simulink model "test_diff"  (R2020b)
settings: Solver=FixedStepAuto  StartTime=0.0  StopTime=20  FixedStep=0.1  RelTol=1e-3
model workspace (MATLAB code in the model file):
  | R = 0.266;
  | r = 0.04;
  | a = 0.3;
  | b = 0.8;
  | anpha1 = -pi/2;
  | anpha2 = pi/6;
  | anpha3 = 5*pi/6;
  | m1 = 0.42;
  | m2 = 0.2;
  | m3 = 0.75;
  | IAy = m1*a*a/3;
  | g = 9.81;
settings Model: OrderedModelArguments=off  Creator=ShiningDanyang  LastModifiedBy=ShiningDanyang

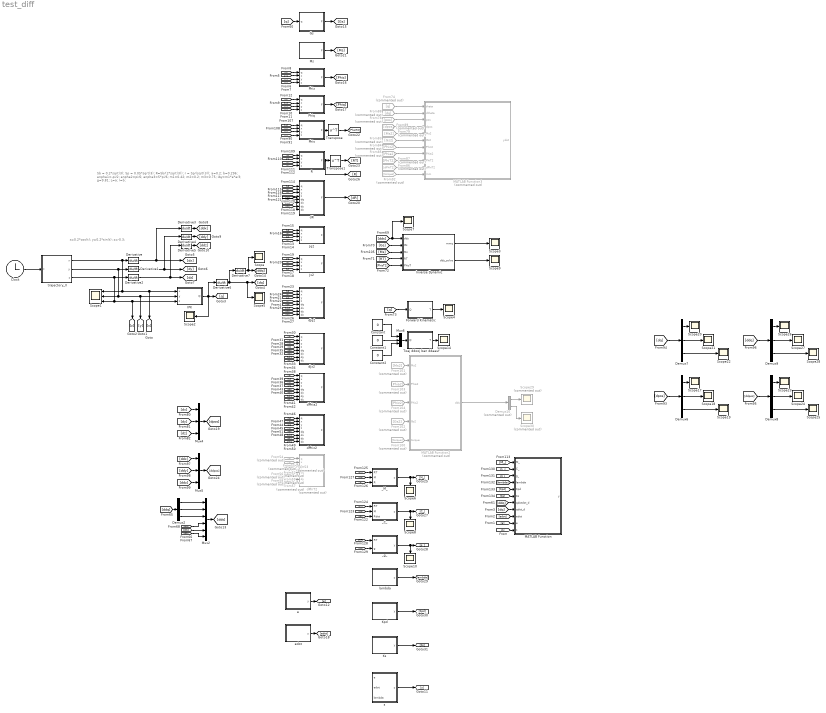
== system test_diff ==
  note: x=0.2*cos(t); y=0.2*sin(t); z=-0.3;
  note: Sb = 0.2*sqrt(3); Sp = 0.05*sqrt(3);
      | R=Sb/(2*sqrt(3)); r = Sp/(sqrt(3));
      | a=0.2; b=0.296;
      | anpha1=-pi/2; anpha2=pi/6; anpha3=5*pi/6;
      | m1=0.42; m2=0.2; m3=0.75;
      | IAy=m1*a*a/3; g=9.81;
      | L=a; l=b;
  Clock : Clock
  Constant : Constant  Value=0
  Constant1 : Constant  Value=0
  Constant2 : Constant  Value=0
  Demux10 : Demux  Commented=on  Outputs=2
  Demux{2,6..9} (5 alike) : Demux  Outputs=3
  Derivative{,1..7} (8 alike) : Derivative
  Forward Kinematic : MATLAB Function  TreatAsAtomicUnit=on
  From100 : From  Commented=on  GotoTag=torque
  From101 : From  Commented=on  GotoTag=Ms2
  From102 : From  Commented=on  GotoTag=Gs2
  From103 : From  Commented=on  GotoTag=Phia2
  From104 : From  Commented=on  GotoTag=Phiz2
  From52 : From  Commented=on  GotoTag=y
  From53 : From  Commented=on  GotoTag=z
  From54 : From  Commented=on  GotoTag=q
  From55 : From  Commented=on  GotoTag=x
  From56 : From  Commented=on  GotoTag=dx
  From57 : From  Commented=on  GotoTag=dy
  From58 : From  Commented=on  GotoTag=dz
  From59 : From  Commented=on  GotoTag=dq
  From74 : From  Commented=on  GotoTag=q
  From78 : From  Commented=on  GotoTag=pos
  From79 : From  Commented=on  GotoTag=Ms2
  From83 : From  Commented=on  GotoTag=Gs2
  From84 : From  Commented=on  GotoTag=Phiz2
  From85 : From  Commented=on  GotoTag=Phia2
  From86 : From  Commented=on  GotoTag=dPhiT2
  From87 : From  Commented=on  GotoTag=PhiT2
  From88 : From  Commented=on  GotoTag=dq
  From89 : From  Commented=on  GotoTag=dpos
  From92 : From  Commented=on  GotoTag=torque
  Gs : MATLAB Function  TreatAsAtomicUnit=on
  IPK : MATLAB Function  TreatAsAtomicUnit=on
  "Inverse Dynamic " : MATLAB Function  TreatAsAtomicUnit=on
  Jq2 : MATLAB Function  TreatAsAtomicUnit=on
  Jx2 : MATLAB Function  TreatAsAtomicUnit=on
  Kpd : MATLAB Function  TreatAsAtomicUnit=on
  Ks : MATLAB Function  TreatAsAtomicUnit=on
  MATLAB Function : MATLAB Function  TreatAsAtomicUnit=on
  MATLAB Function2 : MATLAB Function  Commented=on  TreatAsAtomicUnit=on
  MATLAB Function3 : MATLAB Function  Commented=on  TreatAsAtomicUnit=on
  Ms : MATLAB Function  TreatAsAtomicUnit=on
  Mux2 : Mux  Inputs=6
  Mux4 : Mux  Inputs=3
  Mux5 : Mux  Inputs=3
  Mux6 : Mux  Inputs=3
  Phiq : MATLAB Function  TreatAsAtomicUnit=on
  Phis : MATLAB Function  TreatAsAtomicUnit=on
  Phiz : MATLAB Function  TreatAsAtomicUnit=on
  R : MATLAB Function  TreatAsAtomicUnit=on
  Scope{,2..10,14,17..28} (23 alike) : Scope
  Scope1 : Scope  NumInputPorts=3
  Scope29 : Scope  Commented=on
  Scope30 : Scope  Commented=on
  Toaj ddooj ban ddaauf : MATLAB Function  TreatAsAtomicUnit=on
  Transpose : Math  Operator=transpose  SaturateOnIntegerOverflow=on
  Transpose1 : Math  Operator=transpose  SaturateOnIntegerOverflow=on
  _C_ : MATLAB Function  TreatAsAtomicUnit=on
  _M_ : MATLAB Function  TreatAsAtomicUnit=on
  _g_ : MATLAB Function  TreatAsAtomicUnit=on
  dJq2 : MATLAB Function  TreatAsAtomicUnit=on
  dJx2 : MATLAB Function  TreatAsAtomicUnit=on
  dPhiT2 : MATLAB Function  Commented=on  TreatAsAtomicUnit=on
  dPhia2 : MATLAB Function  TreatAsAtomicUnit=on
  dPhiz2 : MATLAB Function  TreatAsAtomicUnit=on
  dR : MATLAB Function  TreatAsAtomicUnit=on
  e : MATLAB Function  TreatAsAtomicUnit=on
  edot : MATLAB Function  TreatAsAtomicUnit=on
  lambda : MATLAB Function  TreatAsAtomicUnit=on
  s : MATLAB Function  TreatAsAtomicUnit=on
  trajectory_X : MATLAB Function  TreatAsAtomicUnit=on
  wires:
  Clock/1 -> trajectory_X/1(t)
  trajectory_X/1(x) -> IPK/1(x), [x], Scope1/1, Derivative/1
  trajectory_X/2(y) -> IPK/2(y), [y], Scope1/2, Derivative1/1
  trajectory_X/3(z) -> IPK/3(z), [z], Scope1/3, Derivative2/1
  Derivative2/1 -> [dz], Derivative5/1
  Derivative1/1 -> [dy], Derivative4/1
  Derivative/1 -> [dx], Derivative3/1
  IPK/1(Q) -> Scope2/1, [q], Derivative6/1
  Derivative6/1 -> Derivative7/1, Scope5/1, [dq]
  [q] -> Phiz/1(q)
  [x] -> Phiz/2(x)
  [y] -> Phiz/3(y)
  [z] -> Phiz/4(z)
  [z] -> Phiq/4(z)
  [y] -> Phiq/3(y)
  [x] -> Phiq/2(x)
  [q] -> Phiq/1(q)
  [y] -> Jx2/3(y)
  [q] -> Jx2/1(q)
  [x] -> Jx2/2(x)
  [z] -> Jx2/4(z)
  [q] -> dJq2/1(q)
  [x] -> dJq2/2(x)
  [y] -> dJq2/3(y)
  [z] -> dJq2/4(z)
  [dx] -> dJq2/6(dx)
  [dy] -> dJq2/7(dy)
  [dz] -> dJq2/8(dz)
  [dq] -> dJq2/5(dq)
  [z] -> dJx2/4(z)
  [dx] -> dJx2/6(dx)
  [x] -> dJx2/2(x)
  [dq] -> dJx2/5(dq)
  [y] -> dJx2/3(y)
  [dy] -> dJx2/7(dy)
  [dz] -> dJx2/8(dz)
  [q] -> dJx2/1(q)
  [z] -> dPhia2/4(z)
  [dx] -> dPhia2/6(dx)
  [x] -> dPhia2/2(x)
  [dq] -> dPhia2/5(dq)
  [y] -> dPhia2/3(y)
  [dy] -> dPhia2/7(dy)
  [dz] -> dPhia2/8(dz)
  [q] -> dPhia2/1(q)
  [z] -> dPhiz2/4(z)
  [dx] -> dPhiz2/6(dx)
  [x] -> dPhiz2/2(x)
  [dq] -> dPhiz2/5(dq)
  [y] -> dPhiz2/3(y)
  [dy] -> dPhiz2/7(dy)
  [dz] -> dPhiz2/8(dz)
  [q] -> dPhiz2/1(q)
  From53/1 -> dPhiT2/4(z)
  From56/1 -> dPhiT2/6(dx)
  From55/1 -> dPhiT2/2(x)
  From59/1 -> dPhiT2/5(dq)
  From52/1 -> dPhiT2/3(y)
  From57/1 -> dPhiT2/7(dy)
  From58/1 -> dPhiT2/8(dz)
  From54/1 -> dPhiT2/1(q)
  [q] -> Gs/1(q)
  Derivative3/1 -> [ddx]
  Derivative4/1 -> [ddy]
  Derivative5/1 -> [ddz]
  [ddx] -> Mux2/4
  [ddy] -> Mux2/5
  [ddq] -> Demux2/1
  Mux2/1 -> [dds]
  Demux2/1 -> Mux2/1
  Demux2/3 -> Mux2/3
  [ddz] -> Mux2/6
  Demux2/2 -> Mux2/2
  Derivative7/1 -> Scope/1, [ddq]
  [dds] -> Scope7/1, "Inverse Dynamic "/1(dds)
  Gs/1(F) -> [Gs]
  [Gs] -> "Inverse Dynamic "/2(Gs)
  Phiz/1(F) -> [Phiz]
  Phiq/1(F) -> [Phiq]
  "Inverse Dynamic "/1(mmq) -> Scope3/1
  [q] -> Forward Kinematic/1(Q)
  Forward Kinematic/1(T) -> Scope4/1
  [dz] -> Mux4/3
  [dx] -> Mux4/1
  Mux4/1 -> [dpos]
  [dy] -> Mux4/2
  Ms/1(F) -> [Ms]
  [q] -> Phis/1(q)
  [dpos] -> Demux6/1
  Demux6/1 -> Scope17/1
  Demux6/2 -> Scope18/1
  Demux6/3 -> Scope19/1
  [dq] -> Demux7/1
  Demux7/1 -> Scope20/1
  Demux7/2 -> Scope21/1
  Demux7/3 -> Scope22/1
  Demux9/3 -> Scope28/1
  Demux9/1 -> Scope26/1
  [ddpos] -> Demux8/1
  [ddq] -> Demux9/1
  Demux8/1 -> Scope23/1
  Demux9/2 -> Scope27/1
  Demux8/2 -> Scope24/1
  Demux8/3 -> Scope25/1
  [ddz] -> Mux5/3
  [ddy] -> Mux5/2
  Mux5/1 -> [ddpos]
  [ddx] -> Mux5/1
  From100/1 -> MATLAB Function2/5(torque)
  From101/1 -> MATLAB Function2/1(Ms2)
  From102/1 -> MATLAB Function2/4(Gs2)
  From103/1 -> MATLAB Function2/2(Phia2)
  From104/1 -> MATLAB Function2/3(Phiz2)
  [Ms] -> "Inverse Dynamic "/3(Ms)
  MATLAB Function2/1(dds) -> Demux10/1
  Demux10/1 -> Scope29/1
  Demux10/2 -> Scope30/1
  From74/1 -> MATLAB Function3/1(theta)
  From78/1 -> MATLAB Function3/3(pos)
  From79/1 -> MATLAB Function3/5(Ms2)
  From83/1 -> MATLAB Function3/6(Gs2)
  From84/1 -> MATLAB Function3/7(Phiz2)
  From85/1 -> MATLAB Function3/8(Phia2)
  From86/1 -> MATLAB Function3/10(dPhiT2)
  From87/1 -> MATLAB Function3/9(PhiT2)
  From88/1 -> MATLAB Function3/2(dtheta)
  From89/1 -> MATLAB Function3/4(dpos)
  From92/1 -> MATLAB Function3/11(mm)
  [y] -> Phis/3(y)
  [z] -> Phis/4(z)
  [x] -> Phis/2(x)
  Transpose/1 -> [PhisT2]
  Phis/1(F) -> Transpose/1
  [q] -> R/1(q)
  [x] -> R/2(x)
  [z] -> R/4(z)
  [y] -> R/3(y)
  R/1(F) -> [R], Transpose1/1
  Transpose1/1 -> [RT]
  [RT] -> "Inverse Dynamic "/4(RT)
  "Inverse Dynamic "/2(dds_solve) -> Scope9/1
  [PhisT2] -> "Inverse Dynamic "/5(PhisT)
  [y] -> Jq2/3(y)
  [q] -> Jq2/1(q)
  [z] -> Jq2/4(z)
  [x] -> Jq2/2(x)
  Mux6/1 -> Toaj ddooj ban ddaauf/1(Q)
  Constant/1 -> Mux6/1
  Constant1/1 -> Mux6/2
  Constant2/1 -> Mux6/3
  Toaj ddooj ban ddaauf/1(T) -> Scope14/1
  [q] -> dR/1(q)
  [y] -> dR/3(y)
  [x] -> dR/2(x)
  [z] -> dR/4(z)
  [dq] -> dR/5(dq)
  [dx] -> dR/6(dx)
  [dy] -> dR/7(dy)
  [dz] -> dR/8(dz)
  dR/1(F) -> [dR]
  [dR] -> _C_/3(Rdot)
  [Ms] -> _C_/2(M)
  [RT] -> _C_/1(RT)
  [RT] -> _M_/1(RT)
  [R] -> _M_/3(R)
  [Ms] -> _M_/2(M)
  [RT] -> _g_/1(RT)
  [Gs] -> _g_/2(g)
  _M_/1(y) -> [M_], Scope6/1
  _C_/1(y) -> Scope8/1, [C_]
  _g_/1(y) -> Scope10/1, [g_]
  [M_] -> MATLAB Function/1(M_)
  [C_] -> MATLAB Function/2(C_)
  [g_] -> MATLAB Function/3(g_)
  lambda/1(y) -> [lambda]
  [lambda] -> MATLAB Function/4(lambda)
  Kpd/1(y) -> [Kpd]
  [Kpd] -> MATLAB Function/5(Kpd)
  Ks/1(y) -> [Ks]
  [Ks] -> MATLAB Function/6(Ks)
  s/1(y) -> [s]
  [s] -> MATLAB Function/11(s)
  e/1(y) -> [e]
  edot/1(y) -> [edot]
  [e] -> MATLAB Function/10(e)
  [edot] -> MATLAB Function/9(edot)
  [dq] -> MATLAB Function/8(qdot_d)
  [ddq] -> MATLAB Function/7(qdotdot_d)

== matlab function test_diff/dPhia2 ==
  data: q input; F output; x input; y input; z input; dq input; dx input; dy input; dz input
function F = dPhia2(q, x, y, z, dq, dx, dy, dz)
% global R r a b anpha1 anpha2 anpha3 m1 m2 m3 IAy g
Sb = 0.2*sqrt(3); Sp = 0.05*sqrt(3);
R=Sb/(2*sqrt(3)); r = Sp/(sqrt(3));
a=0.2; b=0.296; 
anpha1=-pi/2; anpha2=pi/6; anpha3=5*pi/6;
m1=0.42; m2=0.2; m3=0.75; IAy=m1*a*a/3; g=9.81;
% global a R r anpha1 anpha2 anpha3
F = [
    2*a*(cos(q(1))*(R-r)*dq(1)-cos(anpha1)*(cos(q(1))*x*dq(1)+sin(q(1))*dx)-sin(anpha1)*(cos(q(1))*y*dq(1)+sin(q(1))*dy)+sin(q(1))*z*dq(1)-cos(q(1))*dz),0,0,
    0,2*a*(cos(q(2))*(R-r)*dq(2)-cos(anpha2)*(cos(q(2))*x*dq(2)+sin(q(2))*dx)-sin(anpha2)*(cos(q(2))*y*dq(2)+sin(q(2))*dy)+sin(q(2))*z*dq(2)-cos(q(2))*dz),0,
    0,0,2*a*(cos(q(3))*(R-r)*dq(3)-cos(anpha3)*(cos(q(3))*x*dq(3)+sin(q(3))*dx)-sin(anpha3)*(cos(q(3))*y*dq(3)+sin(q(3))*dy)+sin(q(3))*z*dq(3)-cos(q(3))*dz)
];

== matlab function test_diff/dPhiT2 ==
  data: q input; F output; x input; y input; z input; dq input; dx input; dy input; dz input
function F = dPhiT2(q, x, y, z, dq, dx, dy, dz)
% global R r a b anpha1 anpha2 anpha3 m1 m2 m3 IAy g
Sb = 0.2*sqrt(3); Sp = 0.05*sqrt(3);
R=Sb/(2*sqrt(3)); r = Sp/(sqrt(3));
a=0.2; b=0.296; 
anpha1=-pi/2; anpha2=pi/6; anpha3=5*pi/6;
m1=0.42; m2=0.2; m3=0.75; IAy=m1*a*a/3; g=9.81;
% global R r anpha1 anpha2 anpha3 a b
F = [
    dPhia2(q,x,y,z,dq,dx,dy,dz), dPhiz2(q,x,y,z,dq,dx,dy,dz)
]';

== matlab function test_diff/dPhiz2 ==
  data: q input; F output; x input; y input; z input; dq input; dx input; dy input; dz input
function F = dPhiz2(q, x, y, z, dq, dx, dy, dz)
% global R r a b anpha1 anpha2 anpha3 m1 m2 m3 IAy g
Sb = 0.2*sqrt(3); Sp = 0.05*sqrt(3);
R=Sb/(2*sqrt(3)); r = Sp/(sqrt(3));
a=0.2; b=0.296; 
anpha1=-pi/2; anpha2=pi/6; anpha3=5*pi/6;
m1=0.42; m2=0.2; m3=0.75; IAy=m1*a*a/3; g=9.81;
% global a anpha1 anpha2 anpha3
F = [
    2*(-a*cos(anpha1)*sin(q(1))*dq(1)-dx),-2*(a*sin(anpha1)*sin(q(1))*dq(1)+dy),-2*(a*cos(q(1))*dq(1)+dz),
    2*(-a*cos(anpha2)*sin(q(2))*dq(2)-dx),-2*(a*sin(anpha2)*sin(q(2))*dq(2)+dy),-2*(a*cos(q(2))*dq(2)+dz),
    2*(-a*cos(anpha3)*sin(q(3))*dq(3)-dx),-2*(a*sin(anpha3)*sin(q(3))*dq(3)+dy),-2*(a*cos(q(3))*dq(3)+dz)
];

== matlab function test_diff/Gs ==
  data: q input; F output
function F = Gs(q)
Sb = 0.2*sqrt(3); Sp = 0.05*sqrt(3);
R=Sb/(2*sqrt(3)); r = Sp/(sqrt(3));
a=0.2; b=0.296; 
anpha1=-pi/2; anpha2=pi/6; anpha3=5*pi/6;
m1=0.42; m2=0.2; m3=0.75; IAy=m1*a*a/3; g=9.81;

F = [
    -a*g*(0.5*m1+m2)*cos(q(1));
    -a*g*(0.5*m1+m2)*cos(q(2));
    -a*g*(0.5*m1+m2)*cos(q(3));
    0;
    0;
    (m3+3*m2)*g
    ];

== matlab function test_diff/Ms ==
  data: F output
function F = Ms()
Sb = 0.2*sqrt(3); Sp = 0.05*sqrt(3);
R=Sb/(2*sqrt(3)); r = Sp/(sqrt(3));
a=0.2; b=0.296; 
anpha1=-pi/2; anpha2=pi/6; anpha3=5*pi/6;
m1=0.42; m2=0.2; m3=0.75; IAy=m1*a*a/3; g=9.81;

F = [
    IAy+m2*a^2,          0,          0,       0,          0,          0;
             0, IAy+m2*a^2,          0,       0,          0,          0;
             0,          0, IAy+m2*a^2,       0,          0,          0;
             0,          0,          0, m3+3*m2,          0,          0;
             0,          0,          0,       0,    m3+3*m2,          0;
             0,          0,          0,       0,          0,    m3+3*m2
    ];
%IAy = I1y (trong taif lieeuj)
%m2 = mb (trong taif lieeuj)
%m3 = mP (trong taif lieeuj)

== matlab function test_diff/Inverse Dynamic  ==
  data: dds input; mmq output; Gs input; Ms input; RT input; dds_solve output; PhisT input
function [mmq, dds_solve]   = fcn(dds, Gs, Ms, RT, PhisT)
Sb = 0.2*sqrt(3); Sp = 0.05*sqrt(3);
R=Sb/(2*sqrt(3)); r = Sp/(sqrt(3));
a=0.2; b=0.296; 
anpha1=-pi/2; anpha2=pi/6; anpha3=5*pi/6;
m1=0.42; m2=0.2; m3=0.75; IAy=m1*a*a/3; g=9.81;

mmq = RT*Ms*dds + RT*Gs;

% dds_solve = 0;
mm = [mmq; 0; 0; 0];
lambda = PhisT\(mm - Ms*dds - Gs);
% disp(lambda);
% disp(size(lambda));
dds_solve = Ms\(mm - PhisT*lambda - Gs);
%     mmt=((Ms2*dds+Gs2))';
%     mm = [mmt(:,1), mmt(:,2), mmt(:,3)];

== matlab function test_diff/Forward Kinematic ==
  data: Q input; T output

% Nguyen Thinh 16CDT2
% Nguyen Quoc Thanh Giao 16CDT1
% 01/09/2019
%Ham tinh dong hoc thuan (FPK)
function T  = FPK_V2(Q)
%param
% Can 5 thong so 
% chieu dai canh tay L, chieu dai khau chap hanh cuoi l, chieu dai canh tam
% giac co dinh sB, chieu dai canh tam giac di dong sP.
% Thong so vi tri can tinh T=[x,y,z]
% Thong so goc quay Q=[q1,q2,q3]
%Chuyen tu do sang radian
% q1=(Q(1)*pi)/180;
% q2=(Q(2)*pi)/180;
% q3=(Q(3)*pi)/180;
q1 = Q(1);
q2 = Q(2);
q3 = Q(3);
%Cac thong so co ban cua delta robot
L=0.2; %Chieu dai canh tay lon
l=0.296; %Chieu dai canh tay nho
Sb = 0.2*sqrt(3); Sp = 0.05*sqrt(3);
% Thong so dung trong tinh toan
Wb=((sqrt(3)/6)*Sb);
Wp=(sqrt(3)/6)*Sp;
Ub=(sqrt(3)/3)*Sb;
Up=(sqrt(3)/3)*Sp;
% Dat cac bien a,b,c de dua he phuong trinh dong hoc thuan ve dang
% x^2 + (y+a+l.cos(q1))^2 + (z + l.sin(q1))^2 = l^2
% (X + b - (Sqrt(3)/2).l.cos(q2) )^2 + (Y + C - (1/2).l.cos(q2))^2 + ( Z + L.sin(q2) )^2 = l^2
% (X - b + (Sqrt(3)/2).l.cos(q3) )^2 + (Y + C - (1/2).l.cos(q3))^2 + ( Z + L.sin(q3) )^2 = l^2
%...........................
a=Wb-Up;
b=(Sp/2)-(sqrt(3)/2)*Wb;
c=Wp-Wb/2;
%...........................
% Dua he phuong trinh ve dang giao diem 3 mat cau
% Cac bien Xi,Yi,Zi voi i=1,2,3 la toa do cua tam 3 mat cau
% Cac bien Ri voi i=1,2,3 la ban kinh 3 mat cau
%.............................
X1=0;
Y1=-a-(L*cos(q1));
Z1=-L*sin(q1);
X2=(sqrt(3)/2)*L*cos(q2)-b;
Y2=((1/2)*L*cos(q2)) - c;
Z2= -L*sin(q2);
X3=-(sqrt(3)/2)*L*cos(q3)+b;
Y3=((1/2)*L*cos(q3)) - c;
Z3= -L*sin(q3);
R1=l;
R2=l;
R3=l;
%...........................
% Dua he giao diem 3 mat cau ve dang:
% a11.x + a12.y + a13.z = b1
% a21.x + a22.y + a23.z = b2
%...........................
a11=2*(X3-X1);
a12=2*(Y3-Y1);
a13=2*(Z3-Z1);
a21=2*(X3-X2);
a22=2*(Y3-Y2);
a23=2*(Z3-Z2);
b1=(R1^2)-(R3^2)-(X1^2)-(Y1^2)-(Z1^2)+(X3^2)+(Y3^2)+(Z3^2);
b2=(R2^2)-(R3^2)-(X2^2)-(Y2^2)-(Z2^2)+(X3^2)+(Y3^2)+(Z3^2);
%...........................
%Kiem tra cac diem ki di
if ((a13==0)||(a23==0))
% Giai theo phu luc B
% [A].[B]=[C] voi
% [A] = [m,n; p,q] ; [X]=[x,y] ; [C]= [k, t]
m = 2*(X3-X1);
n = 2*(Y3-Y1);
p = 2*(X3-X2);
q = 2*(Y3-Y2);
k = X3^2 + Y3^2 - X1^2 -Y1^2;
t = X3^2 + Y3^2 - X2^2 -Y2^2;
[A] = [m,n;p,q] ;
[B]=[;]; 
[C]= [k;t];
[B] = [A]\[C];
Zn=Z1;
x1=B(1);
x2=x1;
x=x1;
y1=B(2);
y2=y1;
y=y1;
% Giai phuong trinh bac 2 tim z
z1 = ((2*Zn) + ( sqrt((-2*Zn)^2 - 4*(Zn^2 - R1^2 + (x - X1)^2 + (y-Y1)^2 )) ))/2;
z2 = ((2*Zn) - ( sqrt((-2*Zn)^2 - 4*(Zn^2 - R1^2 + (x - X1)^2 + (y-Y1)^2 )) ))/2;
else
    % Rut x theo y ( x=f(y)= a4.y + a5 )
% Voi
a1=(a11/a13)-(a21/a23);
a2=(a12/a13)-(a22/a23);
a3=(b2/a23)-(b1/a13);
a4= -a2/a1;
a5= -a3/a1;

%........................
% Rut z theo y z = a6.y + a7
% Voi
a6= (-a21*a4-a22)/a23;
a7= (b2-a21*a5)/a23;
%....................
% Dua ve phuong trinh bac 2 theo y: y = a.y^2 + b.y + c
% Voi 
a=(a4^2)+(a6^2)+1;
b=2*a4*(a5-X1)-2*Y1+2*a6*(a7-Z1);
c=a5*(a5-2*X1)+a7*(a7-2*Z1)+X1^2+Y1^2+Z1^2-R1^2;
%.......................
% Tim nghiem y
y1=(-b+(sqrt(b*b-4*a*c)))/(2*a);
y2=(-b-(sqrt(b*b-4*a*c)))/(2*a);
%........................
% Tinh x,z theo y
x1=a4*y1+a5;
x2=a4*y2+a5;
z1=a6*y1+a7;
z2=a6*y2+a7;
%..........................
end
...........................
T1=[x1,y1,z1];
T2=[x2,y2,z2];
% Loai nghiem z duong 
if (z1<=0)
T=T1;    
else
 T=T2;   
end

== matlab function test_diff/IPK ==
  data: x input; Q output; y input; z input
%% IPK: Ham tinh dong hoc nguoc robot delta.
%% Dau vao la vector vi tri [x,y,z], dau ra la vi tri
%% goc quay [q1,q2,q3]
function Q  = IPK(x,y,z)

 %% Khai bao cac hang so su dung
 Pi = 3.141;
 esilon = 10e-8;

 %% Khai bao thong so cua robot
Sb = 0.2*sqrt(3); Sp = 0.05*sqrt(3);
R=Sb/(2*sqrt(3)); r = Sp/(sqrt(3));
a=0.2; b=0.296; 
anpha1=-pi/2; anpha2=pi/6; anpha3=5*pi/6;
m1=0.42; m2=0.2; m3=0.75; IAy=m1*a*a/3; g=9.81;
L=a;
l=b;
 h = 0.131; %% chieu rong canh tay hinh binh hanh
 Ub = (sqrt(3) / 3) * Sb;
 Up = (sqrt(3) / 3) * Sp;
 Wb = (sqrt(3) / 6) * Sb;
 Wp = (sqrt(3) / 6) * Sp;

 %% Khai bao cac he so trong tinh toan
 a = (-(Up)+Wb);
 b = ((Sp / 2) - ((sqrt(3)) / 2)* Wb);
 c = (Wp - (Wb / 2));

 %% Ma tran chua thong so cua phuong trinh dong hoc nguoc
 E = zeros(1,3);
 F = zeros(1,3);
 G = zeros(1,3);
 Q = zeros(1,3);
 %% Phuong trinh dong hoc nguoc duoc dua ve dang
 %% Fi.Sin(Qi) + Ei.cos(Qi) + Gi = 0 voi:
 E(1) = (2 * L * (y + a));
 E(2) = (-L * (sqrt(3) * ((x + b)) + y + c));
 E(3) = (L * (sqrt(3) * ((x - b)) - y - c));
 F(1) = (2 * z * L);
 F(2) = 2 * z * L;
 F(3) = 2 * z * L;
 G(1) = x * x + y * y + z * z + a * a + L * L + 2 * y * a - l * l;
 G(2) = x * x + y * y + z * z + b * b + c * c + L * L + 2 * (x * b + y * c) - l * l;
 G(3) = x * x + y * y + z * z + b * b + c * c + L * L + 2 * (-(x * b) + y * c) - l * l;

 %% Kiem tra cac toa do vo nghiem.
 for i = 1:3
    if (( E(i)^2 + F(i)^2 - G(i)^2 ) < 0)

%          fprintf('Khong tim duoc nghiem dong co thu %d \n',i);
        disp('Khoong timf dduocwj nghieemj ddoongj cow thws');
        disp(i);
    else
        t1 = ( -F(i) + sqrt( E(i)^2 + F(i)^2 - G(i)^2 ))/( G(i) - E(i));
        t2 = ( -F(i) - sqrt( E(i)^2 + F(i)^2 - G(i)^2 ))/( G(i) - E(i));
        q11 = 2*atan(t1);
        q12 = 2*atan(t2);
        if abs(q11)>abs(q12)
%             Q(i) = (q12*180)/pi;
            Q(i) = q12;
        else
%             Q(i) = (q11*180)/pi;
            Q(i) = q11;
        end
     end
end

== matlab function test_diff/MATLAB Function3 ==
  data: theta input; dtheta input; ydot output; pos input; dpos input; Ms2 input; Gs2 input; Phiz2 input; Phia2 input; PhiT2 input; dPhiT2 input; mm input
function ydot=xvdot(theta, dtheta, pos, dpos, Ms2, Gs2, Phiz2, Phia2, PhiT2, dPhiT2, mm)
% global R r L1 L2 alpha1 alpha2 alpha3 m1 m2 m3 Ix Iy Iz I2x I2y I2z g
%Dau vao 1
Sb = 0.2*sqrt(3); Sp = 0.05*sqrt(3);
R=Sb/(2*sqrt(3)); r = Sp/(sqrt(3));
a=0.2; b=0.296; 
anpha1=-pi/2; anpha2=pi/6; anpha3=5*pi/6;
m1=0.42; m2=0.2; m3=0.75; IAy=m1*a*a/3; g=9.81;
% cac he so on dinh
alpha=1/0.001; beta=sqrt(2)/0.001; %chinh xac cao thoi gian lau
%alpha=100; beta=100*sqrt(2);
q=theta;
dq=dtheta';
x=pos(1); y=pos(2); z=pos(3);
dx=dpos(1); dy=dpos(2); dz=dpos(3);
s=[q(1),q(2),q(3),x,y,z]';
ds=[dq(1),dq(2),dq(3),dx,dy,dz]';
% Vec to momen dieu khien
u1=mm(1); u2=mm(2); u3=mm(3);
u=[u1,u2,u3,0,0,0]';
% Tinh ma tran M
M=Ms2;
% Tính ma tran C
% C=Cs(q,dq);
C=0;
% Tinh ma tran Gs
G=Gs2;
% Tinh ma tran R
Q=[eye(3,3);-inv(Phiz2)*Phia2];
% tinh ma tran Phi_s la dao ham cua f theo s
Phi=PhiT2'; % PhiT la ma tran da chuyen vi;
% Tinh dao ham theo t cua ma tran PhiT
dPhi=dPhiT2';
H=pos;
F11=Phi*ds;
% Vec to p1
p1=u-C*ds-G;
% Vec to p3 co them on dinh hoa Baungart
p3=-dPhi*ds-2*alpha*Phi*ds-beta*beta*H; %+F2; %-2*alpha*Phi*ds+beta*beta*F;
% Tinh ma tran D
D=[Q'*M;Phi];
dds = (Q'*M)\(Q'*(u-G));
% dds=inv(D)*[Q'*p1;p3];
ydot=dds;
% disp(size(ydot));

== matlab function test_diff/Phis ==
  data: q input; F output; x input; y input; z input
function F = Phis(q, x, y, z)
Sb = 0.2*sqrt(3); Sp = 0.05*sqrt(3);
R=Sb/(2*sqrt(3)); r = Sp/(sqrt(3));
a=0.2; b=0.296; 
anpha1=-pi/2; anpha2=pi/6; anpha3=5*pi/6;
m1=0.42; m2=0.2; m3=0.75; IAy=m1*a*a/3; g=9.81;

q1 = q(1);
q2 = q(2);
q3 = q(3);
F = [
    2*a*(sin(q1)*(R-r)-cos(anpha1)*sin(q1)*x-sin(anpha1)*sin(q1)*y-cos(q1)*z), 0,                                                                         0;
    0,                                                                         2*a*(sin(q2)*(R-r)-cos(anpha2)*sin(q2)*x-sin(anpha2)*sin(q2)*y-cos(q2)*z), 0;
    0,                                                                         0,                                                                         2*a*(sin(q3)*(R-r)-cos(anpha3)*sin(q3)*x-sin(anpha3)*sin(q3)*y-cos(q3)*z);
    2*(cos(anpha1)*(R-r)+a*cos(anpha1)*cos(q1)-x),                             2*(cos(anpha2)*(R-r)+a*cos(anpha2)*cos(q2)-x),                             2*(cos(anpha3)*(R-r)+a*cos(anpha3)*cos(q3)-x);
    2*(sin(anpha1)*(R-r)+a*sin(anpha1)*cos(q1)-y),                             2*(sin(anpha2)*(R-r)+a*sin(anpha2)*cos(q2)-y),                             2*(sin(anpha3)*(R-r)+a*sin(anpha3)*cos(q3)-y);
    2*(z+a*sin(q1)),                                                           2*(z+a*sin(q2)),                                                           2*(z+a*sin(q3))
    ]';

== matlab function test_diff/MATLAB Function2 ==
  data: Ms2 input; dds output; Phia2 input; Phiz2 input; Gs2 input; torque input
function dds = fcn(Ms2, Phia2, Phiz2, Gs2, torque)
% Q = [eye(3); -inv(Phiz2)*Phia2];
% disp(size(Q'));
invPz=inv(Phiz2);
Pa=Phia2;
Q=[eye(3,3);-invPz*Pa]; % Q <=> R(trong taif lieeuj)
mm=torque;
% dds = mm'/(Q'*Ms2 + Q'*Gs2);
dds = Ms2\(Q'\mm' - Gs2);
% disp(size(dds))

== matlab function test_diff/R ==
  data: q input; F output; x input; y input; z input
function F = R(q, x, y, z)
Sb = 0.2*sqrt(3); Sp = 0.05*sqrt(3);
R=Sb/(2*sqrt(3)); r = Sp/(sqrt(3));
a=0.2; b=0.296; 
anpha1=-pi/2; anpha2=pi/6; anpha3=5*pi/6;
m1=0.42; m2=0.2; m3=0.75; IAy=m1*a*a/3; g=9.81;

q1 = q(1);
q2 = q(2);
q3 = q(3);

F = [
    eye(3);
    -inv(Phiz(q, x, y, z))*Phiq(q, x, y, z)
    ];

== matlab function test_diff/Jq2 ==
  data: q input; F output; x input; y input; z input
function F = Jq2(q, x, y, z)
% global R r a b anpha1 anpha2 anpha3 m1 m2 m3 IAy g
Sb = 0.2*sqrt(3); Sp = 0.05*sqrt(3);
R=Sb/(2*sqrt(3)); r = Sp/(sqrt(3));
a=0.2; b=0.296; 
anpha1=-pi/2; anpha2=pi/6; anpha3=5*pi/6;
m1=0.42; m2=0.2; m3=0.75; IAy=m1*a*a/3; g=9.81;
% global R r a anpha1 anpha2 anpha3
F = [
    2*a*(cos(anpha1)*(R-r)+a*cos(anpha1)*cos(q(1))-x)*cos(anpha1)*sin(q(1))+2*a*(sin(anpha1)*(R-r)+a*sin(anpha1)*cos(q(1))-y)*sin(anpha1)*sin(q(1))-2*a*(a*sin(q(1))+z)*cos(q(1)),0,0,
    0,2*a*(cos(anpha2)*(R-r)+a*cos(anpha2)*cos(q(2))-x)*cos(anpha2)*sin(q(2))+2*a*(sin(anpha2)*(R-r)+a*sin(anpha2)*cos(q(2))-y)*sin(anpha2)*sin(q(2))-2*a*(a*sin(q(2))+z)*cos(q(2)),0,
    0,0,2*a*(cos(anpha3)*(R-r)+a*cos(anpha3)*cos(q(3))-x)*cos(anpha3)*sin(q(3))+2*a*(sin(anpha3)*(R-r)+a*sin(anpha3)*cos(q(3))-y)*sin(anpha3)*sin(q(3))-2*a*(a*sin(q(3))+z)*cos(q(3))
];

== matlab function test_diff/_M_ ==
  data: RT input; y output; M input; R input
function y = fcn(RT,M,R)

y = RT*M*R;
% disp(size(y))

== matlab function test_diff/_C_ ==
  data: RT input; y output; M input; Rdot input
function y = fcn(RT,M,Rdot)

y = RT*M*Rdot;
disp(size(y))

== matlab function test_diff/_g_ ==
  data: RT input; y output; g input
function y = fcn(RT, g)

y = RT*g;

== matlab function test_diff/dR ==
  data: q input; F output; x input; y input; z input; dq input; dx input; dy input; dz input
function F = R(q, x, y, z, dq, dx, dy, dz)
Sb = 0.2*sqrt(3); Sp = 0.05*sqrt(3);
R=Sb/(2*sqrt(3)); r = Sp/(sqrt(3));
a=0.2; b=0.296; 
anpha1=-pi/2; anpha2=pi/6; anpha3=5*pi/6;
m1=0.42; m2=0.2; m3=0.75; IAy=m1*a*a/3; g=9.81;

q1 = q(1);
q2 = q(2);
q3 = q(3);

F = [
    eye(3);
%     -inv(Phiz(q, x, y, z))*Phiq(q, x, y, z)
    inv(Phiz(q, x, y, z))*dPhiz(q, x, y, z, dq, dx, dy, dz)*inv(Phiz(q, x, y, z))*Phiq(q, x, y, z) - inv(Phiz(q, x, y, z))*dPhiq(q, x, y, z, dq, dx, dy, dz)
    ];

== matlab function test_diff/trajectory_X ==
  data: x output; t input; y output; z output
function [x, y, z] = fcn(t)
% tf = 1;
%start at [0; 0; -0.1585]
% if(t<=2)
%     x = 0;
%     y = 0;
%     z = -0.1585-t*0.0707;
% elseif(t<=4 && t>2)
%     x = (t-2)/10;
%     y = 0;
%     z = -0.3;
% else
    x=0.2*cos(t-4);
    y=0.2*sin(t-4);
    z=-0.3;
% end

== matlab function test_diff/MATLAB Function ==
  data: M_ input; y output; C_ input; g_ input; lambda input; Kpd input; Ks input; qdotdot_d input; qdot_d input; edot input; e input; s input
function y = fcn(M_, C_, g_, lambda, Kpd, Ks, qdotdot_d, qdot_d, edot, e, s)

y = M_*qdotdot_d' + C_*qdot_d' + g_ - M_*lambda*edot - C_*lambda*e - Kpd*s - Ks*sign(s);

== matlab function test_diff/lambda ==
  data: y output
function y = fcn()

y = diag([3,3,3]);

== matlab function test_diff/Kpd ==
  data: y output
function y = fcn()

y = diag([4,4,4]);

== matlab function test_diff/Ks ==
  data: y output
function y = fcn()

y = diag([5,5,5]);

== matlab function test_diff/s ==
  data: e input; y output; edot input; lambda input
function y = fcn(e, edot, lambda)

y = e + lambda*edot;

== matlab function test_diff/e ==
  data: y output
function y = fcn()

y = [1;2;3];

== matlab function test_diff/edot ==
  data: y output
function y = fcn()

y = [1;2;3];

== matlab function test_diff/Phiz ==
  data: q input; F output; x input; y input; z input
function F = Phiz(q, x, y, z)
Sb = 0.2*sqrt(3); Sp = 0.05*sqrt(3);
R=Sb/(2*sqrt(3)); r = Sp/(sqrt(3));
a=0.2; b=0.296; 
anpha1=-pi/2; anpha2=pi/6; anpha3=5*pi/6;
m1=0.42; m2=0.2; m3=0.75; IAy=m1*a*a/3; g=9.81;

q1 = q(1);
q2 = q(2);
q3 = q(3);
F = [
    2*(cos(anpha1)*(R-r)+a*cos(anpha1)*cos(q1)-x), 2*(cos(anpha2)*(R-r)+a*cos(anpha2)*cos(q2)-x), 2*(cos(anpha3)*(R-r)+a*cos(anpha3)*cos(q3)-x);
    2*(sin(anpha1)*(R-r)+a*sin(anpha1)*cos(q1)-y), 2*(sin(anpha2)*(R-r)+a*sin(anpha2)*cos(q2)-y), 2*(sin(anpha3)*(R-r)+a*sin(anpha3)*cos(q3)-y);
    2*(z+a*sin(q1)),                               2*(z+a*sin(q2)),                               2*(z+a*sin(q3))
    ]';

== matlab function test_diff/Phiq ==
  data: q input; F output; x input; y input; z input
function F = Phiq(q, x, y, z)
Sb = 0.2*sqrt(3); Sp = 0.05*sqrt(3);
R=Sb/(2*sqrt(3)); r = Sp/(sqrt(3));
a=0.2; b=0.296; 
anpha1=-pi/2; anpha2=pi/6; anpha3=5*pi/6;
m1=0.42; m2=0.2; m3=0.75; IAy=m1*a*a/3; g=9.81;

q1 = q(1);
q2 = q(2);
q3 = q(3);
F = [
    2*a*(sin(q1)*(R-r)-cos(anpha1)*sin(q1)*x-sin(anpha1)*sin(q1)*y-cos(q1)*z), 0,                                                                         0;
    0,                                                                         2*a*(sin(q2)*(R-r)-cos(anpha2)*sin(q2)*x-sin(anpha2)*sin(q2)*y-cos(q2)*z), 0;
    0,                                                                         0,                                                                         2*a*(sin(q3)*(R-r)-cos(anpha3)*sin(q3)*x-sin(anpha3)*sin(q3)*y-cos(q3)*z)
    ]';

== matlab function test_diff/Toaj ddooj ban ddaauf ==
  data: Q input; T output

% Nguyen Thinh 16CDT2
% Nguyen Quoc Thanh Giao 16CDT1
% 01/09/2019
%Ham tinh dong hoc thuan (FPK)
function T  = FPK_V2(Q)
%param
% Can 5 thong so 
% chieu dai canh tay L, chieu dai khau chap hanh cuoi l, chieu dai canh tam
% giac co dinh sB, chieu dai canh tam giac di dong sP.
% Thong so vi tri can tinh T=[x,y,z]
% Thong so goc quay Q=[q1,q2,q3]
%Chuyen tu do sang radian
% q1=(Q(1)*pi)/180;
% q2=(Q(2)*pi)/180;
% q3=(Q(3)*pi)/180;
q1 = Q(1);
q2 = Q(2);
q3 = Q(3);
%Cac thong so co ban cua delta robot
L=0.2; %Chieu dai canh tay lon
l=0.296; %Chieu dai canh tay nho
Sb = 0.2*sqrt(3); Sp = 0.05*sqrt(3);
% Thong so dung trong tinh toan
Wb=((sqrt(3)/6)*Sb);
Wp=(sqrt(3)/6)*Sp;
Ub=(sqrt(3)/3)*Sb;
Up=(sqrt(3)/3)*Sp;
% Dat cac bien a,b,c de dua he phuong trinh dong hoc thuan ve dang
% x^2 + (y+a+l.cos(q1))^2 + (z + l.sin(q1))^2 = l^2
% (X + b - (Sqrt(3)/2).l.cos(q2) )^2 + (Y + C - (1/2).l.cos(q2))^2 + ( Z + L.sin(q2) )^2 = l^2
% (X - b + (Sqrt(3)/2).l.cos(q3) )^2 + (Y + C - (1/2).l.cos(q3))^2 + ( Z + L.sin(q3) )^2 = l^2
%...........................
a=Wb-Up;
b=(Sp/2)-(sqrt(3)/2)*Wb;
c=Wp-Wb/2;
%...........................
% Dua he phuong trinh ve dang giao diem 3 mat cau
% Cac bien Xi,Yi,Zi voi i=1,2,3 la toa do cua tam 3 mat cau
% Cac bien Ri voi i=1,2,3 la ban kinh 3 mat cau
%.............................
X1=0;
Y1=-a-(L*cos(q1));
Z1=-L*sin(q1);
X2=(sqrt(3)/2)*L*cos(q2)-b;
Y2=((1/2)*L*cos(q2)) - c;
Z2= -L*sin(q2);
X3=-(sqrt(3)/2)*L*cos(q3)+b;
Y3=((1/2)*L*cos(q3)) - c;
Z3= -L*sin(q3);
R1=l;
R2=l;
R3=l;
%...........................
% Dua he giao diem 3 mat cau ve dang:
% a11.x + a12.y + a13.z = b1
% a21.x + a22.y + a23.z = b2
%...........................
a11=2*(X3-X1);
a12=2*(Y3-Y1);
a13=2*(Z3-Z1);
a21=2*(X3-X2);
a22=2*(Y3-Y2);
a23=2*(Z3-Z2);
b1=(R1^2)-(R3^2)-(X1^2)-(Y1^2)-(Z1^2)+(X3^2)+(Y3^2)+(Z3^2);
b2=(R2^2)-(R3^2)-(X2^2)-(Y2^2)-(Z2^2)+(X3^2)+(Y3^2)+(Z3^2);
%...........................
%Kiem tra cac diem ki di
if ((a13==0)||(a23==0))
% Giai theo phu luc B
% [A].[B]=[C] voi
% [A] = [m,n; p,q] ; [X]=[x,y] ; [C]= [k, t]
m = 2*(X3-X1);
n = 2*(Y3-Y1);
p = 2*(X3-X2);
q = 2*(Y3-Y2);
k = X3^2 + Y3^2 - X1^2 -Y1^2;
t = X3^2 + Y3^2 - X2^2 -Y2^2;
[A] = [m,n;p,q] ;
[B]=[;]; 
[C]= [k;t];
[B] = [A]\[C];
Zn=Z1;
x1=B(1);
x2=x1;
x=x1;
y1=B(2);
y2=y1;
y=y1;
% Giai phuong trinh bac 2 tim z
z1 = ((2*Zn) + ( sqrt((-2*Zn)^2 - 4*(Zn^2 - R1^2 + (x - X1)^2 + (y-Y1)^2 )) ))/2;
z2 = ((2*Zn) - ( sqrt((-2*Zn)^2 - 4*(Zn^2 - R1^2 + (x - X1)^2 + (y-Y1)^2 )) ))/2;
else
    % Rut x theo y ( x=f(y)= a4.y + a5 )
% Voi
a1=(a11/a13)-(a21/a23);
a2=(a12/a13)-(a22/a23);
a3=(b2/a23)-(b1/a13);
a4= -a2/a1;
a5= -a3/a1;

%........................
% Rut z theo y z = a6.y + a7
% Voi
a6= (-a21*a4-a22)/a23;
a7= (b2-a21*a5)/a23;
%....................
% Dua ve phuong trinh bac 2 theo y: y = a.y^2 + b.y + c
% Voi 
a=(a4^2)+(a6^2)+1;
b=2*a4*(a5-X1)-2*Y1+2*a6*(a7-Z1);
c=a5*(a5-2*X1)+a7*(a7-2*Z1)+X1^2+Y1^2+Z1^2-R1^2;
%.......................
% Tim nghiem y
y1=(-b+(sqrt(b*b-4*a*c)))/(2*a);
y2=(-b-(sqrt(b*b-4*a*c)))/(2*a);
%........................
% Tinh x,z theo y
x1=a4*y1+a5;
x2=a4*y2+a5;
z1=a6*y1+a7;
z2=a6*y2+a7;
%..........................
end
...........................
T1=[x1,y1,z1];
T2=[x2,y2,z2];
% Loai nghiem z duong 
if (z1<=0)
T=T1;    
else
 T=T2;   
end
% disp(T);

== matlab function test_diff/Jx2 ==
  data: q input; F output; x input; y input; z input
function F = Jx2(q, x, y, z)
% global R r a b anpha1 anpha2 anpha3 m1 m2 m3 IAy g
Sb = 0.2*sqrt(3); Sp = 0.05*sqrt(3);
R=Sb/(2*sqrt(3)); r = Sp/(sqrt(3));
a=0.2; b=0.296; 
anpha1=-pi/2; anpha2=pi/6; anpha3=5*pi/6;
m1=0.42; m2=0.2; m3=0.75; IAy=m1*a*a/3; g=9.81;
% global a R r anpha1 anpha2 anpha3
F = [
    2*(cos(anpha1)*(R-r)+a*cos(anpha1)*cos(q(1))-x),2*(sin(anpha1)*(R-r)+a*sin(anpha1)*cos(q(1))-y),-2*(a*sin(q(1))+z);
    2*(cos(anpha2)*(R-r)+a*cos(anpha2)*cos(q(2))-x),2*(sin(anpha2)*(R-r)+a*sin(anpha2)*cos(q(2))-y),-2*(a*sin(q(2))+z);
    2*(cos(anpha3)*(R-r)+a*cos(anpha3)*cos(q(3))-x),2*(sin(anpha3)*(R-r)+a*sin(anpha3)*cos(q(3))-y),-2*(a*sin(q(3))+z)
];

== matlab function test_diff/dJq2 ==
  data: q input; F output; x input; y input; z input; dq input; dx input; dy input; dz input
function F = dJq2(q, x, y, z, dq, dx, dy, dz)
% global R r a b anpha1 anpha2 anpha3 m1 m2 m3 IAy g
Sb = 0.2*sqrt(3); Sp = 0.05*sqrt(3);
R=Sb/(2*sqrt(3)); r = Sp/(sqrt(3));
a=0.2; b=0.296; 
anpha1=-pi/2; anpha2=pi/6; anpha3=5*pi/6;
m1=0.42; m2=0.2; m3=0.75; IAy=m1*a*a/3; g=9.81;
% global R r a anpha1 anpha2 anpha3
F = [
    2*a*cos(anpha1)*(cos(anpha1)*(R-r)+a*cos(anpha1)*cos(q(1))-x)*cos(q(1))*dq(1)+2*a*cos(anpha1)*sin(q(1))*(-a*cos(anpha1)*sin(q(1))*dq(1)-dx)+2*a*sin(anpha1)*((sin(anpha1)*(R-r)+a*sin(anpha1)*cos(q(1))-y)*cos(q(1))*dq(1)+sin(q(1))*(-a*sin(anpha1)*sin(q(1))*dq(1)-dy))+2*a*(a*sin(q(1))+z)*sin(q(1))*dq(1)-2*a*cos(q(1))*(a*cos(q(1))*dq(1)+dz),0,0,
    0,2*a*cos(anpha2)*(cos(anpha2)*(R-r)+a*cos(anpha2)*cos(q(2))-x)*cos(q(2))*dq(2)+2*a*cos(anpha2)*sin(q(2))*(-a*cos(anpha2)*sin(q(2))*dq(2)-dx)+2*a*sin(anpha2)*((sin(anpha2)*(R-r)+a*sin(anpha2)*cos(q(2))-y)*cos(q(2))*dq(2)+sin(q(2))*(-a*sin(anpha2)*sin(q(2))*dq(2)-dy))+2*a*(a*sin(q(2))+z)*sin(q(2))*dq(2)-2*a*cos(q(2))*(a*cos(q(2))*dq(2)+dz),0,
    0,0,2*a*cos(anpha3)*(cos(anpha3)*(R-r)+a*cos(anpha3)*cos(q(3))-x)*cos(q(3))*dq(3)+2*a*cos(anpha3)*sin(q(3))*(-a*cos(anpha3)*sin(q(3))*dq(3)-dx)+2*a*sin(anpha3)*((sin(anpha3)*(R-r)+a*sin(anpha3)*cos(q(3))-y)*cos(q(3))*dq(3)+sin(q(3))*(-a*sin(anpha3)*sin(q(3))*dq(3)-dy))+2*a*(a*sin(q(3))+z)*sin(q(3))*dq(3)-2*a*cos(q(3))*(a*cos(q(3))*dq(3)+dz)
];

== matlab function test_diff/dJx2 ==
  data: q input; F output; x input; y input; z input; dq input; dx input; dy input; dz input
function F = dJx2(q, x, y, z, dq, dx,dy, dz)
% global R r a b anpha1 anpha2 anpha3 m1 m2 m3 IAy g
Sb = 0.2*sqrt(3); Sp = 0.05*sqrt(3);
R=Sb/(2*sqrt(3)); r = Sp/(sqrt(3));
a=0.2; b=0.296; 
anpha1=-pi/2; anpha2=pi/6; anpha3=5*pi/6;
m1=0.42; m2=0.2; m3=0.75; IAy=m1*a*a/3; g=9.81;
% global a anpha1 anpha2 anpha3
F = [
    2*(-a*cos(anpha1)*sin(q(1))*dq(1)-dx),2*(-a*sin(anpha1)*sin(q(1))*dq(1)-dy),-2*(a*cos(q(1))*dq(1)+dz);
    2*(-a*cos(anpha2)*sin(q(2))*dq(2)-dx),2*(-a*sin(anpha2)*sin(q(2))*dq(2)-dy),-2*(a*cos(q(2))*dq(2)+dz);
    2*(-a*cos(anpha3)*sin(q(3))*dq(3)-dx),2*(-a*sin(anpha3)*sin(q(3))*dq(3)-dy),-2*(a*cos(q(3))*dq(3)+dz);
];
